simulink model "PID_fourtanks"  (Simulink 7.6)
settings: Solver=ode45  StartTime=0.0  StopTime=inf  RelTol=1e-3
libraries: opclib x5, simulink x2
settings Model: Creator=Administrator  LastModifiedBy=Administrator
settings OptimizationCC: InitFltsAndDblsToZero=on
settings DebuggingCC: StrictBusMsg=Warning

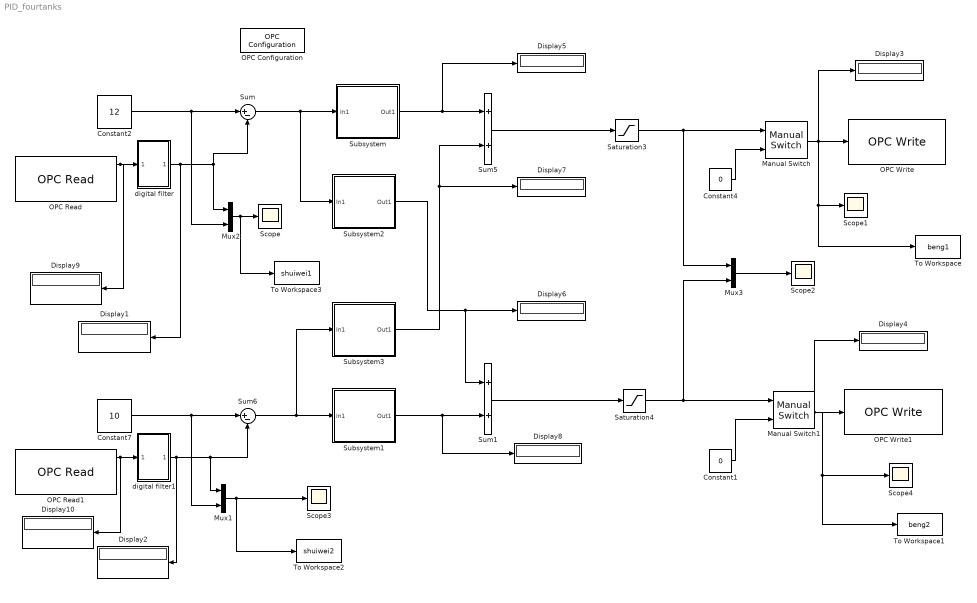
== system PID_fourtanks ==
  Constant1 : Constant  Value=0
  Constant2 : Constant  Value=12
  Constant4 : Constant  Value=0
  Constant7 : Constant  Value=10
  Display{1..10} (10 alike) : Display
  Manual Switch : simulink/Signal Routing/Manual Switch  SystemSampleTime=-1  sw=1  action=0  varsize=off
  Manual Switch1 : simulink/Signal Routing/Manual Switch  SystemSampleTime=-1  sw=1  action=0  varsize=off
  Mux1 : Mux  Inputs=2
  Mux2 : Mux  Inputs=2
  Mux3 : Mux  Inputs=2
  OPC Configuration : opclib/OPC Configuration  opcServers=localhost/OPCServer.WinCC/10  errMissingItems=Error  errReadWrite=Warn  errShutdown=Error  errRTViolation=None  rtEnable=on  speedup=1  showLatency=off  beingUsed=on
  OPC Read : opclib/OPC Read  serverHost=localhost  serverID=OPCServer.WinCC  itemIDs=shuiwei1  readMode=Synchronous (cache)  dataType=double  updateRate=0.01  showQual=on  showTS=on  tsMode=Seconds since start
  OPC Read1 : opclib/OPC Read  serverHost=localhost  serverID=OPCServer.WinCC  itemIDs=shuiwei2  readMode=Synchronous (cache)  dataType=double  updateRate=0.5  showQual=on  showTS=on  tsMode=Seconds since start
  OPC Write : opclib/OPC Write  serverHost=localhost  serverID=OPCServer.WinCC  itemIDs=beng1  writeMode=Synchronous  updateRate=0
  OPC Write1 : opclib/OPC Write  serverHost=localhost  serverID=OPCServer.WinCC  itemIDs=beng2  writeMode=Synchronous  updateRate=0
  Saturation3 : Saturate  UpperLimit=100  LowerLimit=0
  Saturation4 : Saturate  UpperLimit=100  LowerLimit=0
  Scope{,1..4} (5 alike) : Scope
      Scope settings: TimeRange=1000  YMin=0  YMax=30  SaveName=shuiwei1  DataFormat=Array
      Scope1 settings: TimeRange=1000  YMin=82.5  YMax=89.5  SaveName=shuiwei  DataFormat=Array
      Scope2 settings: TimeRange=1000  YMin=40.5  YMax=52  SaveName=ScopeData2
      Scope3 settings: TimeRange=1000  YMin=0  YMax=20  SaveName=shuiwei2  DataFormat=Array
      Scope4 settings: TimeRange=1000  YMin=0  YMax=100  SaveName=shuiwei3  DataFormat=Array
  Subsystem : Subsystem  mask{P=6, I=0.4, D=0, S=0.2}
      mask prompts: P "proporation"; I "integrator"; D "derivative"; S "antigain"
      mask Display: disp('SPID\nControl')
  Subsystem1 : Subsystem  mask{P=5, I=0.4, D=0, S=0.2}
      mask prompts: P "proporation"; I "integrator"; D "derivative"; S "antigain"
      mask Display: disp('SPID\nControl')
  Subsystem2 : Subsystem  mask{P=3, I=0.2, D=0, S=1}
      mask prompts: P "proporation"; I "integrator"; D "derivative"; S "antigain"
      mask Display: disp('SPID\nControl')
  Subsystem3 : Subsystem  mask{P=3, I=0.2, D=0, S=0.2}
      mask prompts: P "proporation"; I "integrator"; D "derivative"; S "antigain"
      mask Display: disp('SPID\nControl')
  Sum : Sum  Inputs=|+-
  Sum1 : Sum
  Sum5 : Sum
  Sum6 : Sum  Inputs=|+-
  To Workspace : ToWorkspace  VariableName=beng1  SampleTime=0.5  SaveFormat=Array
  To Workspace1 : ToWorkspace  VariableName=beng2  SampleTime=0.5  SaveFormat=Array
  To Workspace2 : ToWorkspace  VariableName=shuiwei2  SampleTime=0.5  SaveFormat=Array
  To Workspace3 : ToWorkspace  VariableName=shuiwei1  SampleTime=0.5  SaveFormat=Array
  digital filter : Subsystem
  digital filter1 : Subsystem
  wires:
  Constant2/1 -> Sum/1, Mux2/2
  Sum/1 -> Subsystem/1(In1), Subsystem2/1(In1)
  Subsystem/1(Out1) -> Sum5/1, Display5/1
  Sum5/1 -> Saturation3/1
  Saturation3/1 -> Mux3/1, Manual Switch/1
  Manual Switch/1 -> OPC Write/1, Display3/1, Scope1/1, To Workspace/1
  Constant4/1 -> Manual Switch/2
  Constant7/1 -> Sum6/1, Mux1/2
  Sum6/1 -> Subsystem1/1(In1), Subsystem3/1(In1)
  Sum1/1 -> Saturation4/1
  Saturation4/1 -> Manual Switch1/1, Mux3/2
  Manual Switch1/1 -> OPC Write1/1, Display4/1, Scope4/1, To Workspace1/1
  OPC Read1/1 -> Display10/1, digital filter1/1(In1)
  OPC Read/1 -> Display9/1, digital filter/1(In1)
  Constant1/1 -> Manual Switch1/2
  Subsystem1/1(Out1) -> Sum1/2, Display8/1
  Subsystem2/1(Out1) -> Sum1/1, Display6/1
  Subsystem3/1(Out1) -> Sum5/2, Display7/1
  Mux2/1 -> Scope/1, To Workspace3/1
  Mux1/1 -> Scope3/1, To Workspace2/1
  Mux3/1 -> Scope2/1
  digital filter/1(Out1) -> Display1/1, Mux2/1, Sum/2
  digital filter1/1(Out1) -> Sum6/2, Mux1/1, Display2/1

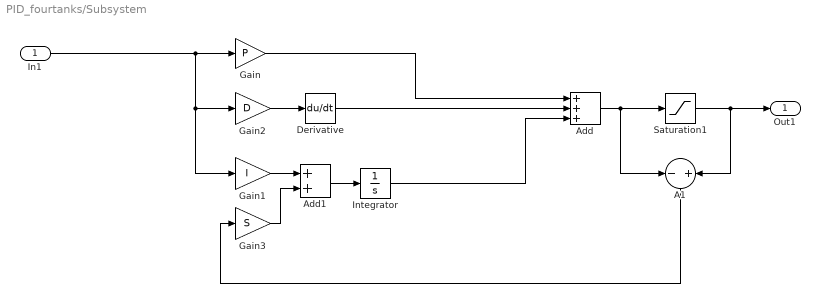
== system PID_fourtanks/Subsystem ==
  In1 : Inport
  A1 : Sum  Inputs=-+
  Add : Sum  Inputs=+++
  Add1 : Sum
  Derivative : Derivative
  Gain : Gain  Gain=P
  Gain1 : Gain  Gain=I
  Gain2 : Gain  Gain=D
  Gain3 : Gain  Gain=S
  Integrator : Integrator
  Saturation1 : Saturate  UpperLimit=75  LowerLimit=0
  Out1 : Outport
  wires:
  In1/1 -> Gain/1, Gain2/1, Gain1/1
  Gain/1 -> Add/1
  Gain2/1 -> Derivative/1
  Add/1 -> Saturation1/1, A1/1
  Derivative/1 -> Add/2
  Integrator/1 -> Add/3
  A1/1 -> Gain3/1
  Gain1/1 -> Add1/1
  Add1/1 -> Integrator/1
  Gain3/1 -> Add1/2
  Saturation1/1 -> Out1/1, A1/2

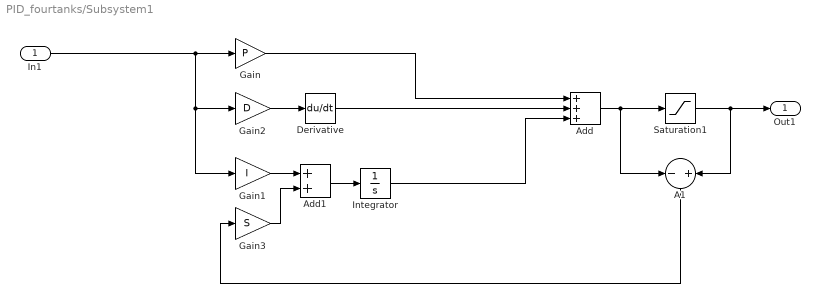
== system PID_fourtanks/Subsystem1 ==
  In1 : Inport
  A1 : Sum  Inputs=-+
  Add : Sum  Inputs=+++
  Add1 : Sum
  Derivative : Derivative
  Gain : Gain  Gain=P
  Gain1 : Gain  Gain=I
  Gain2 : Gain  Gain=D
  Gain3 : Gain  Gain=S
  Integrator : Integrator
  Saturation1 : Saturate  UpperLimit=75  LowerLimit=0
  Out1 : Outport
  wires:
  Saturation1/1 -> A1/2, Out1/1
  Gain3/1 -> Add1/2
  Add1/1 -> Integrator/1
  Gain1/1 -> Add1/1
  A1/1 -> Gain3/1
  Integrator/1 -> Add/3
  Derivative/1 -> Add/2
  Add/1 -> A1/1, Saturation1/1
  Gain2/1 -> Derivative/1
  Gain/1 -> Add/1
  In1/1 -> Gain1/1, Gain2/1, Gain/1

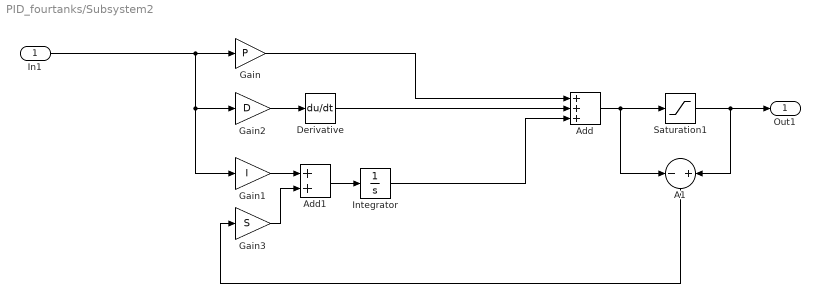
== system PID_fourtanks/Subsystem2 ==
  In1 : Inport
  A1 : Sum  Inputs=-+
  Add : Sum  Inputs=+++
  Add1 : Sum
  Derivative : Derivative
  Gain : Gain  Gain=P
  Gain1 : Gain  Gain=I
  Gain2 : Gain  Gain=D
  Gain3 : Gain  Gain=S
  Integrator : Integrator
  Saturation1 : Saturate  UpperLimit=25  LowerLimit=-25
  Out1 : Outport
  wires:
  Saturation1/1 -> A1/2, Out1/1
  Gain3/1 -> Add1/2
  Add1/1 -> Integrator/1
  Gain1/1 -> Add1/1
  A1/1 -> Gain3/1
  Integrator/1 -> Add/3
  Derivative/1 -> Add/2
  Add/1 -> A1/1, Saturation1/1
  Gain2/1 -> Derivative/1
  Gain/1 -> Add/1
  In1/1 -> Gain1/1, Gain2/1, Gain/1

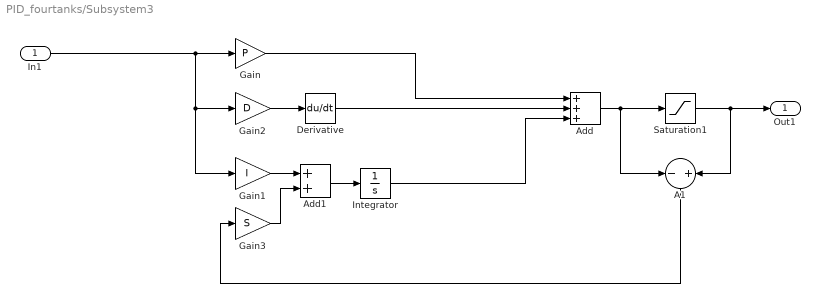
== system PID_fourtanks/Subsystem3 ==
  In1 : Inport
  A1 : Sum  Inputs=-+
  Add : Sum  Inputs=+++
  Add1 : Sum
  Derivative : Derivative
  Gain : Gain  Gain=P
  Gain1 : Gain  Gain=I
  Gain2 : Gain  Gain=D
  Gain3 : Gain  Gain=S
  Integrator : Integrator
  Saturation1 : Saturate  UpperLimit=25  LowerLimit=-25
  Out1 : Outport
  wires:
  In1/1 -> Gain/1, Gain2/1, Gain1/1
  Gain/1 -> Add/1
  Gain2/1 -> Derivative/1
  Add/1 -> Saturation1/1, A1/1
  Derivative/1 -> Add/2
  Integrator/1 -> Add/3
  A1/1 -> Gain3/1
  Gain1/1 -> Add1/1
  Add1/1 -> Integrator/1
  Gain3/1 -> Add1/2
  Saturation1/1 -> Out1/1, A1/2

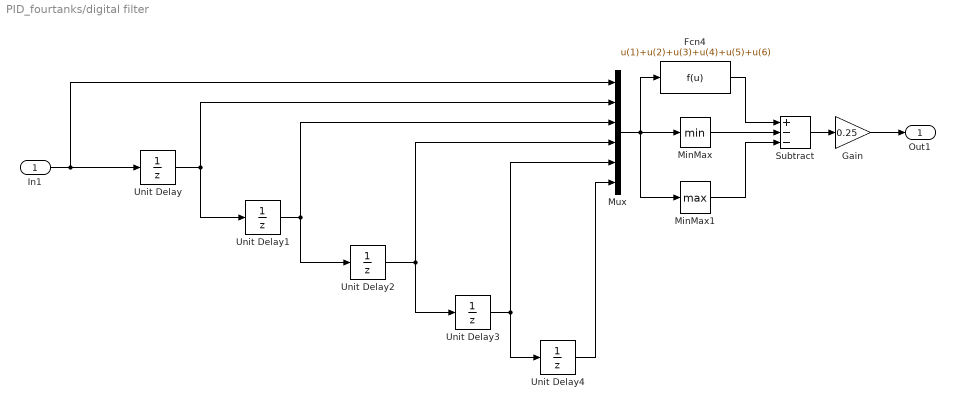
== system PID_fourtanks/digital filter ==
  In1 : Inport
  Fcn4 : Fcn  Expr=u(1)+u(2)+u(3)+u(4)+u(5)+u(6)  SampleTime=0.5
  Gain : Gain  Gain=0.25
  MinMax : MinMax
  MinMax1 : MinMax  Function=max
  Mux : Mux  Inputs=6
  Subtract : Sum  Inputs=+--
  Unit Delay{,1..4} (5 alike) : UnitDelay  SampleTime=0.5
  Out1 : Outport
  wires:
  Unit Delay/1 -> Mux/2, Unit Delay1/1
  Unit Delay1/1 -> Mux/3, Unit Delay2/1
  Unit Delay2/1 -> Mux/4, Unit Delay3/1
  In1/1 -> Unit Delay/1, Mux/1
  Unit Delay3/1 -> Mux/5, Unit Delay4/1
  Mux/1 -> Fcn4/1, MinMax/1, MinMax1/1
  Fcn4/1 -> Subtract/1
  MinMax/1 -> Subtract/2
  MinMax1/1 -> Subtract/3
  Subtract/1 -> Gain/1
  Unit Delay4/1 -> Mux/6
  Gain/1 -> Out1/1

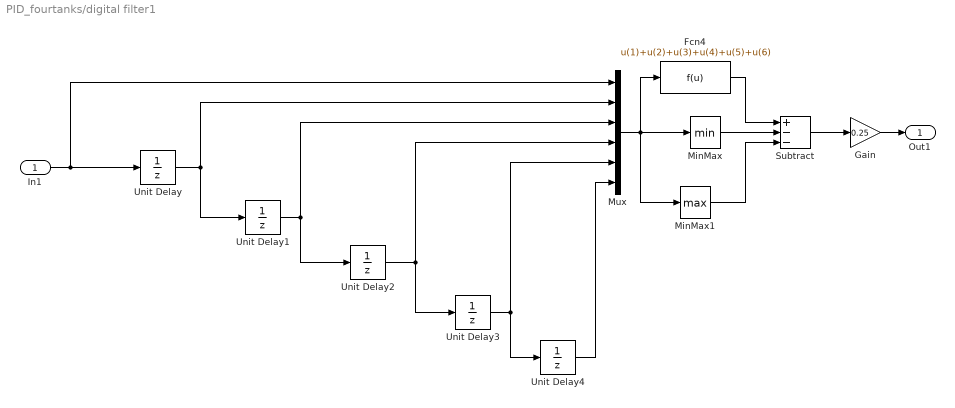
== system PID_fourtanks/digital filter1 ==
  In1 : Inport
  Fcn4 : Fcn  Expr=u(1)+u(2)+u(3)+u(4)+u(5)+u(6)  SampleTime=0.5
  Gain : Gain  Gain=0.25
  MinMax : MinMax
  MinMax1 : MinMax  Function=max
  Mux : Mux  Inputs=6
  Subtract : Sum  Inputs=+--
  Unit Delay{,1..4} (5 alike) : UnitDelay  SampleTime=0.5
  Out1 : Outport
  wires:
  Gain/1 -> Out1/1
  Unit Delay4/1 -> Mux/6
  Subtract/1 -> Gain/1
  MinMax1/1 -> Subtract/3
  MinMax/1 -> Subtract/2
  Fcn4/1 -> Subtract/1
  Mux/1 -> MinMax1/1, MinMax/1, Fcn4/1
  Unit Delay3/1 -> Unit Delay4/1, Mux/5
  In1/1 -> Mux/1, Unit Delay/1
  Unit Delay2/1 -> Unit Delay3/1, Mux/4
  Unit Delay1/1 -> Unit Delay2/1, Mux/3
  Unit Delay/1 -> Unit Delay1/1, Mux/2
